simulink model "integ_gain2_slew"  (Simulink 7.1)
settings: Solver=ode45  StartTime=0.0  StopTime=10.0  RelTol=1e-3
undefined symbols (not defined in the file): alfa, gamma, GBW, INTmax, slew, SR, Ts
settings Model: Creator=yasuda  LastModifiedBy=akira
settings DebuggingCC: SaveWithParameterizedLinksMsg=none
settings GRTTargetCC: TargetFcnLib=ansi_tfl_tmw.mat

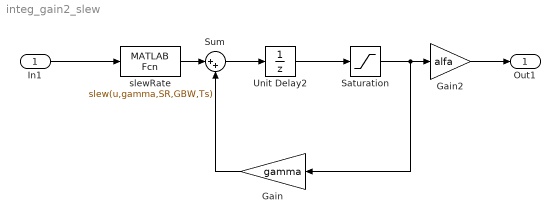
== system integ_gain2_slew ==
  In1 : Inport  OutDataType=sfix(16)  OutScaling=2^0
  Gain : Gain  Orientation=left  Gain=gamma  ParameterDataType=sfix(16)  ParameterScaling=2^0  OutDataType=sfix(16)  OutScaling=2^0
  Gain2 : Gain  Gain=alfa  ParameterDataType=sfix(16)  ParameterScaling=2^0  OutDataType=sfix(16)  OutScaling=2^0
  Saturation : Saturate  UpperLimit=INTmax  LowerLimit=-INTmax
  Sum : Sum  Inputs=|++  OutDataType=sfix(16)  OutScaling=2^0
  Unit Delay2 : UnitDelay  SampleTime=Ts
  slewRate : MATLABFcn  MATLABFcn=slew(u,gamma,SR,GBW,Ts)
  Out1 : Outport  OutDataType=sfix(16)  OutScaling=2^0
  wires:
  Sum/1 -> Unit Delay2/1
  Saturation/1 -> Gain/1, Gain2/1
  Gain/1 -> Sum/2
  In1/1 -> slewRate/1
  slewRate/1 -> Sum/1
  Unit Delay2/1 -> Saturation/1
  Gain2/1 -> Out1/1
